simulink model "radar"  (R2026a)
settings: Solver=FixedStepDiscrete  StopTime=16 * N_pulses * PRI  FixedStep=N_pulses * PRI
PreLoadFcn:
  | run(fullfile(fileparts(which('radar')),'model','radar_params.m'));run(fullfile(fileparts(which('radar')),'model','waveform_params.m'));run(fullfile(fileparts(which('radar')),'model','array_params.m'));
undefined symbols (not defined in the file or in its folder): N_pulses, Nspp, Nspp_receive, PRI
settings Model: Creator=jerem  LastModifiedBy=jerem
settings RTWCC: SystemTargetFile=ert.tlc  GenCodeOnly=on  GenerateMakefile=off  Description=Embedded Coder
settings ERTTargetCC: RootIOFormat=Part of model data structure  GenerateSampleERTMain=on  CodeInterfacePackaging=Reusable function

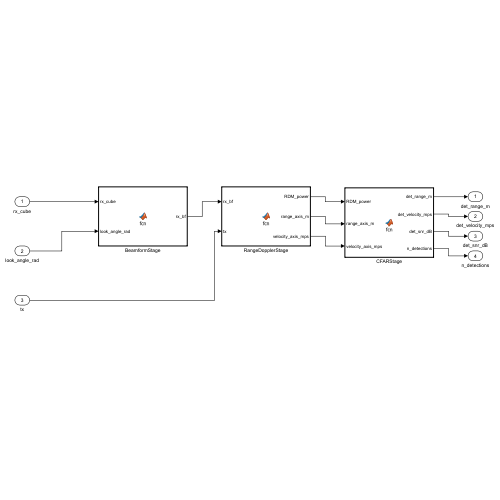
[thumbnail: Simulink's stored preview of the top-level diagram]
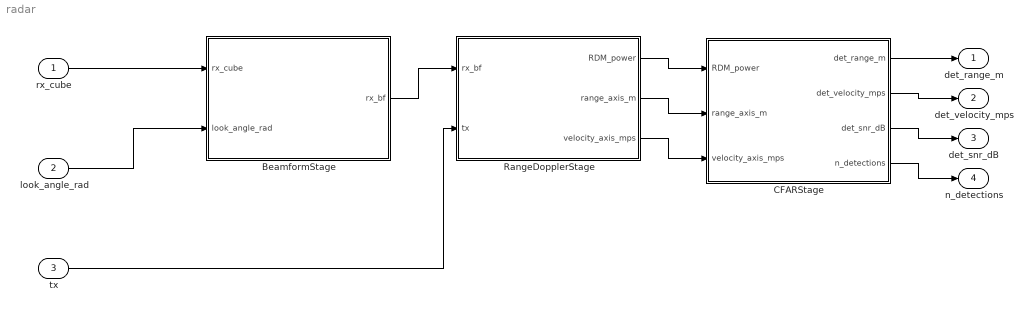
== system radar ==
  rx_cube : Inport  OutDataTypeStr=double  PortDimensions=[Nspp_receive 8 16]  SampleTime=N_pulses * PRI
      settings: SignalType=complex
  look_angle_rad : Inport  Port=2  OutDataTypeStr=double  PortDimensions=1  SampleTime=N_pulses * PRI
  tx : Inport  Port=3  OutDataTypeStr=double  PortDimensions=[Nspp 1]  SampleTime=N_pulses * PRI
      settings: SignalType=complex
  BeamformStage : MATLAB Function  TreatAsAtomicUnit=on
  CFARStage : MATLAB Function  TreatAsAtomicUnit=on
  RangeDopplerStage : MATLAB Function  TreatAsAtomicUnit=on
  det_range_m : Outport
  det_velocity_mps : Outport  Port=2
  det_snr_dB : Outport  Port=3
  n_detections : Outport  Port=4
  wires:
  rx_cube/1 -> BeamformStage/1(rx_cube)
  look_angle_rad/1 -> BeamformStage/2(look_angle_rad)
  BeamformStage/1(rx_bf) -> RangeDopplerStage/1(rx_bf)
  tx/1 -> RangeDopplerStage/2(tx)
  RangeDopplerStage/1(RDM_power) -> CFARStage/1(RDM_power)
  RangeDopplerStage/2(range_axis_m) -> CFARStage/2(range_axis_m)
  RangeDopplerStage/3(velocity_axis_mps) -> CFARStage/3(velocity_axis_mps)
  CFARStage/1(det_range_m) -> det_range_m/1
  CFARStage/2(det_velocity_mps) -> det_velocity_mps/1
  CFARStage/3(det_snr_dB) -> det_snr_dB/1
  CFARStage/4(n_detections) -> n_detections/1

== matlab function radar/RangeDopplerStage ==
  data: rx_bf input; RDM_power output; tx input; range_axis_m output; velocity_axis_mps output
function [RDM_power, range_axis_m, velocity_axis_mps] = fcn(rx_bf, tx)
%#codegen
    fc     = 2.8e9;
    c      = 2.99792458e8;
    lambda = c / fc;
    fs     = 10e6;
    PRI    = 250e-6;
    [RDM, range_axis_m, velocity_axis_mps] = range_doppler(rx_bf, tx, fs, lambda, PRI);
    RDM_power = abs(RDM).^2;
end

== matlab function radar/BeamformStage ==
  data: rx_cube input; rx_bf output; look_angle_rad input
function rx_bf = fcn(rx_cube, look_angle_rad)
%#codegen
    N_el     = 8;
    fc       = 2.8e9;
    c        = 2.99792458e8;
    lambda   = c / fc;
    d        = lambda / 2;
    mvdr_load = 0.001;
    x_elements = ((0:N_el-1) - (N_el-1)/2)' * d;
    [Nspp, ~, N_pulses] = size(rx_cube);
    rx_stacked = reshape(permute(rx_cube, [1 3 2]), [], N_el);
    [~, w_mvdr] = mvdr_beamform(rx_stacked, x_elements, lambda, look_angle_rad, mvdr_load);
    rx_bf = complex(zeros(Nspp, N_pulses));
    for n = 1:N_pulses
        rx_bf(:, n) = rx_cube(:, :, n) * conj(w_mvdr);
    end
end

== matlab function radar/CFARStage ==
  data: RDM_power input; det_range_m output; range_axis_m input; velocity_axis_mps input; det_velocity_mps output; det_snr_dB output; n_detections output
function [det_range_m, det_velocity_mps, det_snr_dB, n_detections] = fcn(RDM_power, range_axis_m, velocity_axis_mps)
%#codegen
    MAX_DETECTIONS = int32(16);
    N_guard_range = 4;  N_train_range = 8;
    N_guard_dop   = 1;  N_train_dop   = 2;
    Pfa           = 1e-6;
    det_mask = cfar_ca(RDM_power, N_guard_range, N_train_range, N_guard_dop, N_train_dop, Pfa);
    det_range_m      = nan(double(MAX_DETECTIONS), 1);
    det_velocity_mps = nan(double(MAX_DETECTIONS), 1);
    det_snr_dB       = nan(double(MAX_DETECTIONS), 1);
    top_p = zeros(double(MAX_DETECTIONS), 1);
    top_r = zeros(double(MAX_DETECTIONS), 1);
    top_d = zeros(double(MAX_DETECTIONS), 1);
    n_found     = int32(0);
    noise_sum   = 0.0;
    noise_count = 0.0;
    [N_r, N_d] = size(RDM_power);
    for r = 1:N_r
        for d = 1:N_d
            p = RDM_power(r, d);
            if det_mask(r, d)
                if n_found < MAX_DETECTIONS
                    n_found = n_found + int32(1);
                    top_p(double(n_found)) = p;
                    top_r(double(n_found)) = r;
                    top_d(double(n_found)) = d;
                else
                    min_val = top_p(1);  min_idx = int32(1);
                    for k = 2:double(MAX_DETECTIONS)
                        if top_p(k) < min_val
                            min_val = top_p(k);  min_idx = int32(k);
                        end
                    end
                    if p > min_val
                        top_p(double(min_idx)) = p;
                        top_r(double(min_idx)) = r;
                        top_d(double(min_idx)) = d;
                    end
                end
            else
                noise_sum   = noise_sum + p;
                noise_count = noise_count + 1.0;
            end
        end
    end
    if noise_count > 0.0
        noise_floor = noise_sum / noise_count;
    else
        noise_floor = eps;
    end
    % Bubble-sort top-K by power descending (K <= 16 so cost is bounded)
    n_used = double(n_found);
    for i = 1 : n_used - 1
        for j = 1 : n_used - i
            if top_p(j) < top_p(j+1)
                t = top_p(j); top_p(j) = top_p(j+1); top_p(j+1) = t;
                t = top_r(j); top_r(j) = top_r(j+1); top_r(j+1) = t;
                t = top_d(j); top_d(j) = top_d(j+1); top_d(j+1) = t;
            end
        end
    end
    for k = 1 : n_used
        det_range_m(k)      = range_axis_m(top_r(k));
        det_velocity_mps(k) = velocity_axis_mps(top_d(k));
        det_snr_dB(k)       = 10 * log10(max(top_p(k), eps) / max(noise_floor, eps));
    end
    n_detections = n_found;
end
